simulink model "GenNewRECurrentRef"  (R2016a)
settings: Solver=FixedStepDiscrete  StartTime=0  StopTime=7  FixedStep=0.001  RelTol=1e-3
values from neighbouring files (symbols this model uses):
  beta = 0.9    [base_model_hybrid_REcurrent_init.m]
  deltaTdes = 0.2    [base_model_hybrid_REcurrent_init.m]
  enableMultiplePlateau = 1    [base_model_hybrid_REcurrent_init.m]
  enableUpdateRefUp = 0    [base_model_hybrid_REcurrent_init.m]
  percent_upgain_newiref = 0.1    [base_model_hybrid_REcurrent_init.m]
  t_end = 2.0    (= 2)    [base_model_hybrid_REcurrent_init.m]
  threshold_time_newiref = 0.02    [base_model_hybrid_REcurrent_init.m]
undefined symbols (not defined in the file or in its folder): cq, pwm, rt2, trigger
libraries: powerlib_extras x1
settings Model: ExtModeTrigDuration=2  Creator=hbaole  LastModifiedBy=mateusz
settings DataIOCC: SaveFormat=Array  SignalLoggingSaveFormat=ModelDataLogs  SaveOutput=off  SignalLogging=off  DSMLogging=off  SignalLoggingName=sigsOut
settings OptimizationCC: DefaultParameterBehavior=Inlined  UseDivisionForNetSlopeComputation=on  UseFloatMulNetSlope=on  InlineInvariantSignals=on  EnhancedBackFolding=on  ExpressionDepthLimit=2147483647  StateBitsets=on  DataBitsets=on  EfficientFloat2IntCast=on  OptimizeModelRefInitCode=on  LifeSpan=1  MaxStackSize=64
settings DebuggingCC: RTPrefix=warning  SaveWithParameterizedLinksMsg=none  UnderspecifiedInitializationDetection=Classic  MergeDetectMultiDrivingBlocksExec=none  MultiTaskDSMMsg=warning  MultiTaskCondExecSysMsg=none  FcnCallInpInsideContextMsg=UseLocalSettings  UnconnectedInputMsg=none  UnconnectedOutputMsg=none  UnconnectedLineMsg=none  StateNameClashWarn=warning
settings HardwareCC: TargetBitPerPointer=64  TargetLongLongMode=on  TargetIntDivRoundTo=Zero  TargetEndianess=LittleEndian  TargetWordSize=64  TargetHWDeviceType=MATLAB Host  ProdEqTarget=off
settings ModelReferenceCC: ModelReferenceNumInstancesAllowed=Single  PropagateSignalLabelsOutOfModel=off
settings SFSimCC: SimParseCustomCode=off
settings RTWCC: SystemTargetFile=ert.tlc  GenCodeOnly=on  TemplateMakefile=ert_default_tmf  GenerateReport=on  RTWVerbose=off  RetainRTWFile=on  Toolchain=MinGW64 v4.x | gmake (64-bit Windows)  BuildConfiguration=Specify  IncludeHyperlinkInReport=on  LaunchReport=on  TargetLang=C++  GenerateTraceInfo=on  GenerateTraceReport=on  GenerateTraceReportSl=on  GenerateTraceReportSf=on  GenerateTraceReportEml=on  CheckMdlBeforeBuild=Warning
settings CodeAppCC: ForceParamTrailComments=on  OperatorAnnotations=on  SimulinkDataObjDesc=on  SFDataObjDesc=on  MATLABFcnDesc=on  InsertBlockDesc=on  MATLABSourceComments=on
settings ERTTargetCC: GenerateSampleERTMain=on  MultiInstanceERTCode=on  CodeInterfacePackaging=C++ class  InlinedParameterPlacement=NonHierarchical  RootIOFormat=Structure reference  ERTCustomFileTemplate=example_file_process.tlc
settings ConfigComp: CovModelRefEnable=Off

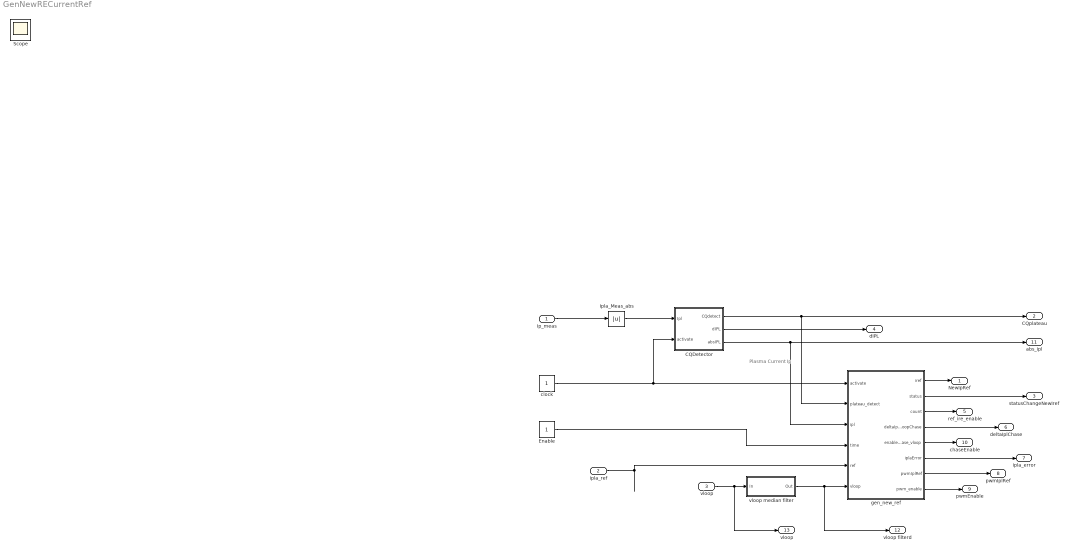
== system GenNewRECurrentRef ==
  note: Plasma Current Ip
  Ip_meas : Inport
  ipla_ref : Inport  Port=2
  vloop : Inport  Port=3
  CQDetector : Subsystem
  Enable : Constant
  Ipla_Meas_abs : Abs
  clock : Constant
  gen_new_ref : Subsystem
  vloop median filter : Subsystem
  NewIpRef : Outport
  CQplateau : Outport  Port=2
  statusChangeNewIref : Outport  Port=3
  dIPL : Outport  Port=4
  ref_ire_enable : Outport  Port=5
  deltaIplChase : Outport  Port=6
  ipla_error : Outport  Port=7
  pwmIplRef : Outport  Port=8
  pwmEnable : Outport  Port=9
  chaseEnable : Outport  Port=10
  abs_ipl : Outport  Port=11
  "vloop filterd " : Outport  Port=12
  "vloop " : Outport  Port=13
  Scope : Scope
  wires:
  CQDetector/1(CQdetect) -> gen_new_ref/2(plateau_detect), CQplateau/1
  CQDetector/2(dIPL) -> dIPL/1
  CQDetector/3(absIPL) -> gen_new_ref/3(ipl), abs_ipl/1
  clock/1 -> CQDetector/2(activate), gen_new_ref/1(activate)
  Ip_meas/1 -> Ipla_Meas_abs/1
  Ipla_Meas_abs/1 -> CQDetector/1(Ipl)
  ipla_ref/1 -> gen_new_ref/5(ref)
  gen_new_ref/1(iref) -> NewIpRef/1
  gen_new_ref/2(status) -> statusChangeNewIref/1
  gen_new_ref/3(count) -> ref_ire_enable/1
  gen_new_ref/4("deltaIplVloopChase ") -> deltaIplChase/1
  gen_new_ref/5(enableChase_vloop) -> chaseEnable/1
  gen_new_ref/6(iplaError) -> ipla_error/1
  gen_new_ref/7(pwmIplRef) -> pwmIplRef/1
  gen_new_ref/8(pwm_enable) -> pwmEnable/1
  Enable/1 -> gen_new_ref/4(time)
  vloop median filter/1(Out) -> "vloop filterd "/1, gen_new_ref/6(vloop)
  vloop/1 -> "vloop "/1, vloop median filter/1(In)

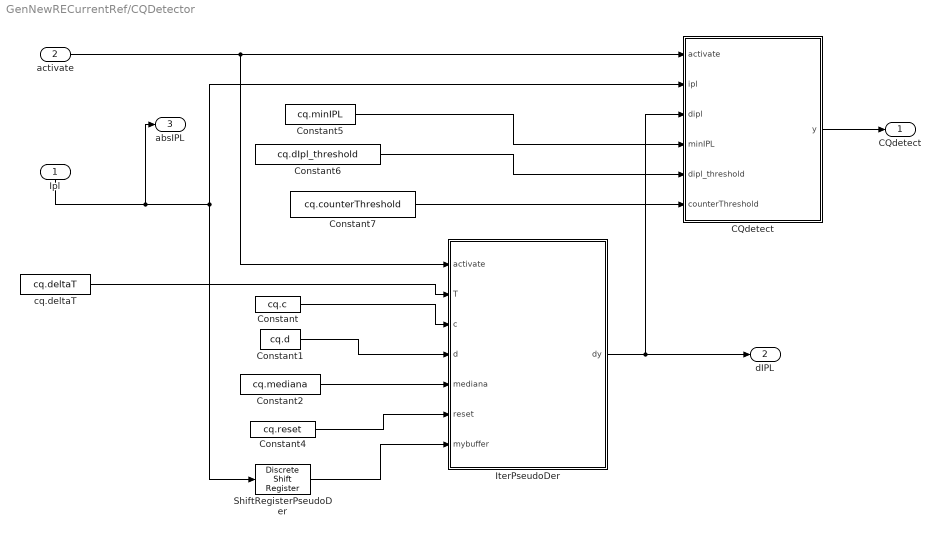
== system GenNewRECurrentRef/CQDetector ==
  Ipl : Inport
  activate : Inport  Port=2
  "CQdetect " : MATLAB Function  TreatAsAtomicUnit=on
  Constant : Constant  Value=cq.c
  Constant1 : Constant  Value=cq.d
  Constant2 : Constant  Value=cq.mediana
  Constant4 : Constant  Value=cq.reset
  Constant5 : Constant  Value=cq.minIPL
  Constant6 : Constant  Value=cq.dIpl_threshold
  Constant7 : Constant  Value=cq.counterThreshold
  IterPseudoDer : MATLAB Function  TreatAsAtomicUnit=on
      settings: RTWSystemCode=Inline
  ShiftRegisterPseudoDer : powerlib_extras/Discrete  Control Blocks/Discrete Shift Register  NSamples=cq.d  InitialValue=0  Ts=rt2.system_period
  cq.deltaT : Constant  Value=cq.deltaT
  CQdetect : Outport
  dIPL : Outport  Port=2
  absIPL : Outport  Port=3
  wires:
  Constant6/1 -> "CQdetect "/5(dipl_threshold)
  activate/1 -> IterPseudoDer/1(activate), "CQdetect "/1(activate)
  Constant5/1 -> "CQdetect "/4(minIPL)
  cq.deltaT/1 -> IterPseudoDer/2(T)
  Constant/1 -> IterPseudoDer/3(c)
  Constant1/1 -> IterPseudoDer/4(d)
  Constant2/1 -> IterPseudoDer/5(mediana)
  Ipl/1 -> absIPL/1, "CQdetect "/2(ipl), ShiftRegisterPseudoDer/1
  "CQdetect "/1(y) -> CQdetect/1
  Constant7/1 -> "CQdetect "/6(counterThreshold)
  IterPseudoDer/1(dy) -> "CQdetect "/3(dipl), dIPL/1
  Constant4/1 -> IterPseudoDer/6(reset)
  ShiftRegisterPseudoDer/1 -> IterPseudoDer/7(mybuffer)

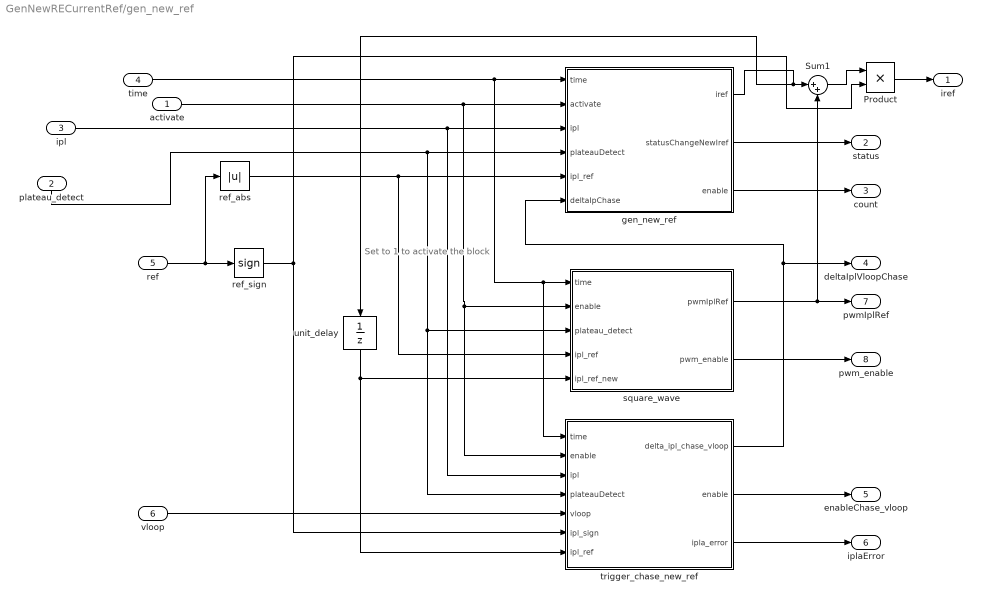
== system GenNewRECurrentRef/gen_new_ref ==
  note: Set to 1 to activate the block
  activate : Inport
  plateau_detect : Inport  Port=2
  ipl : Inport  Port=3
  time : Inport  Port=4
  ref : Inport  Port=5
  vloop : Inport  Port=6
  Product : Product
  Sum1 : Sum  Inputs=|++
  gen_new_ref : Subsystem
  ref_abs : Abs
  ref_sign : Signum
  square_wave : Subsystem
  trigger_chase_new_ref : Subsystem
  unit_delay : UnitDelay  SampleTime=-1
  iref : Outport
  status : Outport  Port=2
  count : Outport  Port=3
  "deltaIplVloopChase " : Outport  Port=4
  enableChase_vloop : Outport  Port=5
  iplaError : Outport  Port=6
  pwmIplRef : Outport  Port=7
  pwm_enable : Outport  Port=8
  wires:
  activate/1 -> trigger_chase_new_ref/2("enable "), square_wave/2("enable "), gen_new_ref/2("activate ")
  ipl/1 -> gen_new_ref/3(ipl), trigger_chase_new_ref/3(ipl)
  ref_abs/1 -> gen_new_ref/5("ipl_ref "), square_wave/4("ipl_ref ")
  time/1 -> square_wave/1(time), trigger_chase_new_ref/1(time), gen_new_ref/1(time)
  ref/1 -> ref_abs/1, ref_sign/1
  ref_sign/1 -> trigger_chase_new_ref/6("ipl_sign "), Product/2
  gen_new_ref/2(statusChangeNewIref) -> status/1
  trigger_chase_new_ref/1(delta_ipl_chase_vloop) -> gen_new_ref/6(deltaIpChase), "deltaIplVloopChase "/1
  gen_new_ref/3(enable) -> count/1
  trigger_chase_new_ref/3(ipla_error) -> iplaError/1
  square_wave/2(pwm_enable) -> pwm_enable/1
  gen_new_ref/1(iref) -> unit_delay/1, Sum1/1
  Sum1/1 -> Product/1
  Product/1 -> iref/1
  vloop/1 -> trigger_chase_new_ref/5(vloop)
  trigger_chase_new_ref/2(enable) -> enableChase_vloop/1
  plateau_detect/1 -> trigger_chase_new_ref/4(plateauDetect), square_wave/3(plateau_detect), gen_new_ref/4(plateauDetect)
  unit_delay/1 -> trigger_chase_new_ref/7("ipl_ref "), square_wave/5(ipl_ref_new)
  square_wave/1(pwmIplRef) -> Sum1/2, pwmIplRef/1

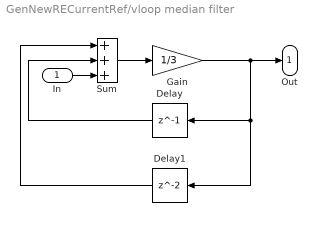
== system GenNewRECurrentRef/vloop median filter ==
  In : Inport
  Delay : Delay  DelayLength=1  InitialCondition=0
  Delay1 : Delay  InitialCondition=0
  Gain : Gain  Gain=1/3
  Sum : Sum  Inputs=|+++  SampleTime=rt2.system_period
  Out : Outport
  wires:
  Gain/1 -> Out/1, Delay1/1, Delay/1
  Delay/1 -> Sum/2
  Sum/1 -> Gain/1
  Delay1/1 -> Sum/1
  In/1 -> Sum/3

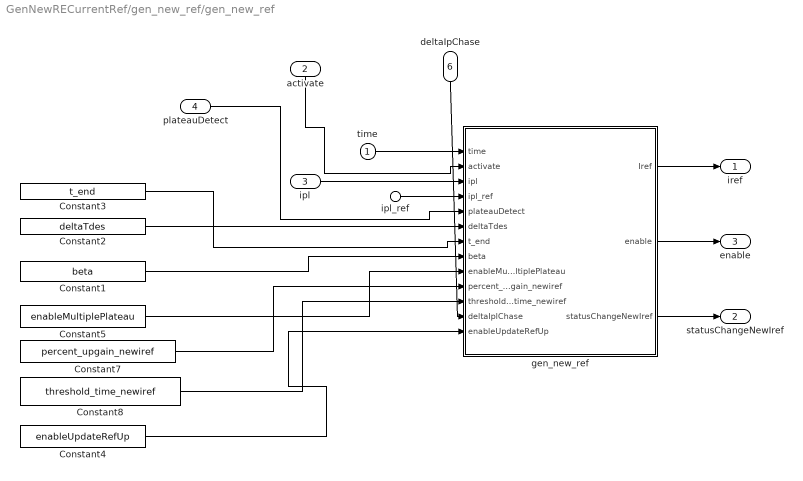
== system GenNewRECurrentRef/gen_new_ref/gen_new_ref ==
  time : Inport
  "activate " : Inport  Port=2
  ipl : Inport  Port=3
  plateauDetect : Inport  Port=4
  "ipl_ref " : Inport  Port=5
  deltaIpChase : Inport  Port=6
  Constant1 : Constant  Value=beta
  Constant2 : Constant  Value=deltaTdes
  Constant3 : Constant  Value=t_end
  Constant4 : Constant  Value=enableUpdateRefUp
  Constant5 : Constant  Value=enableMultiplePlateau
  Constant7 : Constant  Value=percent_upgain_newiref
  Constant8 : Constant  Value=threshold_time_newiref
  gen_new_ref : MATLAB Function  TreatAsAtomicUnit=on
  iref : Outport
  statusChangeNewIref : Outport  Port=2
  enable : Outport  Port=3
  wires:
  plateauDetect/1 -> gen_new_ref/5(plateauDetect)
  gen_new_ref/1(Iref) -> iref/1
  "ipl_ref "/1 -> gen_new_ref/4(ipl_ref)
  gen_new_ref/3(statusChangeNewIref) -> statusChangeNewIref/1
  Constant8/1 -> gen_new_ref/11(threshold_time_newiref)
  Constant7/1 -> gen_new_ref/10(percent_upgain_newiref)
  time/1 -> gen_new_ref/1(time)
  "activate "/1 -> gen_new_ref/2(activate)
  ipl/1 -> gen_new_ref/3(ipl)
  Constant2/1 -> gen_new_ref/6(deltaTdes)
  Constant3/1 -> gen_new_ref/7(t_end)
  gen_new_ref/2(enable) -> enable/1
  Constant5/1 -> gen_new_ref/9(enableMultiplePlateau)
  Constant1/1 -> gen_new_ref/8(beta)
  deltaIpChase/1 -> gen_new_ref/12(deltaIplChase)
  Constant4/1 -> gen_new_ref/13(enableUpdateRefUp)

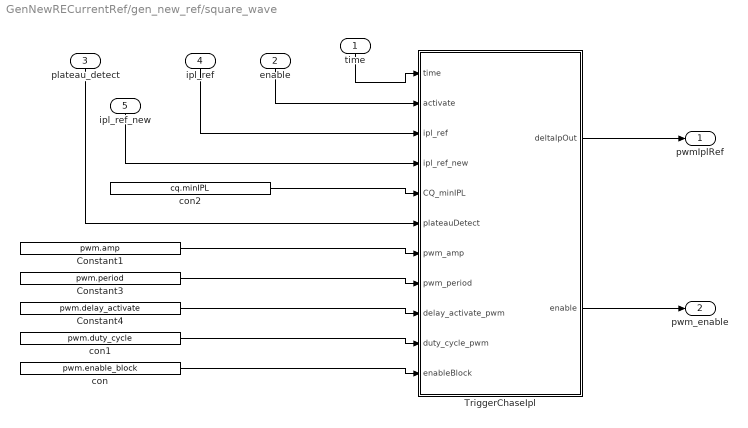
== system GenNewRECurrentRef/gen_new_ref/square_wave ==
  time : Inport
  "enable " : Inport  Port=2
  plateau_detect : Inport  Port=3
  "ipl_ref " : Inport  Port=4
  ipl_ref_new : Inport  Port=5
  Constant1 : Constant  Value=pwm.amp
  Constant3 : Constant  Value=pwm.period
  Constant4 : Constant  Value=pwm.delay_activate
  TriggerChaseIpl : MATLAB Function  TreatAsAtomicUnit=on
  con : Constant  Value=pwm.enable_block
  con1 : Constant  Value=pwm.duty_cycle
  con2 : Constant  Value=cq.minIPL
  pwmIplRef : Outport
  pwm_enable : Outport  Port=2
  wires:
  con/1 -> TriggerChaseIpl/11(enableBlock)
  Constant1/1 -> TriggerChaseIpl/7(pwm_amp)
  TriggerChaseIpl/2(enable) -> pwm_enable/1
  plateau_detect/1 -> TriggerChaseIpl/6(plateauDetect)
  TriggerChaseIpl/1(deltaIpOut) -> pwmIplRef/1
  "enable "/1 -> TriggerChaseIpl/2(activate)
  "ipl_ref "/1 -> TriggerChaseIpl/3(ipl_ref)
  time/1 -> TriggerChaseIpl/1(time)
  Constant3/1 -> TriggerChaseIpl/8(pwm_period)
  Constant4/1 -> TriggerChaseIpl/9(delay_activate_pwm)
  con1/1 -> TriggerChaseIpl/10(duty_cycle_pwm)
  con2/1 -> TriggerChaseIpl/5(CQ_minIPL)
  ipl_ref_new/1 -> TriggerChaseIpl/4(ipl_ref_new)

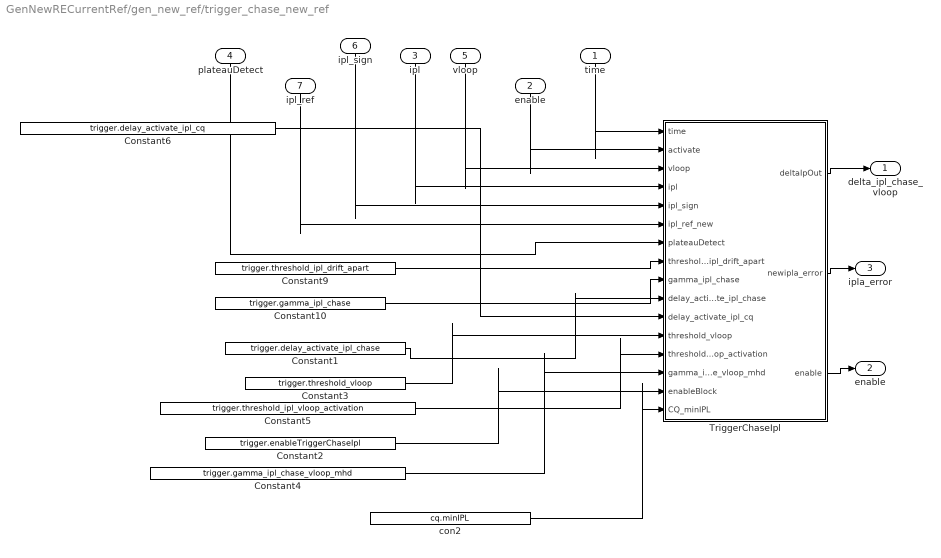
== system GenNewRECurrentRef/gen_new_ref/trigger_chase_new_ref ==
  time : Inport
  "enable " : Inport  Port=2
  ipl : Inport  Port=3
  plateauDetect : Inport  Port=4
  vloop : Inport  Port=5
  "ipl_sign " : Inport  Port=6
  "ipl_ref " : Inport  Port=7
  Constant1 : Constant  Value=trigger.delay_activate_ipl_chase
  Constant10 : Constant  Value=trigger.gamma_ipl_chase
  Constant2 : Constant  Value=trigger.enableTriggerChaseIpl
  Constant3 : Constant  Value=trigger.threshold_vloop
  Constant4 : Constant  Value=trigger.gamma_ipl_chase_vloop_mhd
  Constant5 : Constant  Value=trigger.threshold_ipl_vloop_activation
  Constant6 : Constant  Value=trigger.delay_activate_ipl_cq
  Constant9 : Constant  Value=trigger.threshold_ipl_drift_apart
  TriggerChaseIpl : MATLAB Function  TreatAsAtomicUnit=on
  con2 : Constant  Value=cq.minIPL
  delta_ipl_chase_vloop : Outport
  enable : Outport  Port=2
  ipla_error : Outport  Port=3
  wires:
  ipl/1 -> TriggerChaseIpl/4(ipl)
  time/1 -> TriggerChaseIpl/1(time)
  "ipl_ref "/1 -> TriggerChaseIpl/6(ipl_ref_new)
  Constant10/1 -> TriggerChaseIpl/9(gamma_ipl_chase)
  "enable "/1 -> TriggerChaseIpl/2(activate)
  Constant9/1 -> TriggerChaseIpl/8(threshold_ipl_drift_apart)
  TriggerChaseIpl/1(deltaIpOut) -> delta_ipl_chase_vloop/1
  plateauDetect/1 -> TriggerChaseIpl/7(plateauDetect)
  TriggerChaseIpl/3(enable) -> enable/1
  Constant1/1 -> TriggerChaseIpl/10(delay_activate_ipl_chase)
  Constant2/1 -> TriggerChaseIpl/15(enableBlock)
  TriggerChaseIpl/2(newipla_error) -> ipla_error/1
  vloop/1 -> TriggerChaseIpl/3(vloop)
  "ipl_sign "/1 -> TriggerChaseIpl/5(ipl_sign)
  Constant3/1 -> TriggerChaseIpl/12(threshold_vloop)
  Constant4/1 -> TriggerChaseIpl/14(gamma_ipl_chase_vloop_mhd)
  Constant5/1 -> TriggerChaseIpl/13(threshold_ipl_vloop_activation)
  con2/1 -> TriggerChaseIpl/16(CQ_minIPL)
  Constant6/1 -> TriggerChaseIpl/11(delay_activate_ipl_cq)

== matlab function GenNewRECurrentRef/CQDetector/CQdetect  ==
  data: activate input; ipl input; y output; dipl input; minIPL input; dipl_threshold input; counterThreshold input
function y = cq_detect(activate, ipl, dipl, minIPL, dipl_threshold, counterThreshold)
%% CurrentQuench and RE palteau detection
% INPUT:
%          activate = boolean var for eneabled the alghoritm
%                      0 : active
%                      1 : non active
%           ipl = absolute value of the  plasma current
%           dipl, minIPL, dipl_threshold, counterThreshold : min
%
% OUTPUT:  y in R
%         -1 : detection non active
%          0 : detection active
%          1 : CQ detect
%          2 : RE palteau detect
%%

persistent  startDetection;

if(activate)
    if(isempty(startDetection))
        startDetection = 0;
    end
    
    %STEP1: FIND CQ
    if( ipl >= minIPL)
        
        if( dipl <= dipl_threshold  && mod(startDetection,2)  == 0)
            startDetection = startDetection+1;
        end
        
        if( dipl >=  dipl_threshold  && mod(startDetection,2) == 1)
            startDetection = startDetection+1;
        end
        
    else
        
        if(startDetection > 0)
            startDetection =-1;
        end
        
    end
    
    y = startDetection;
    
else
    y = -2;
end

== matlab function GenNewRECurrentRef/CQDetector/IterPseudoDer ==
  data: activate input; T input; c input; d input; mediana input; reset input; dy output; mybuffer input
function dy = iter_pseudo_der_function(activate,T,c,d,mediana,reset,mybuffer)

 if activate==1 && reset==0
     
     if(mediana==1)
         temp1 = 0;
         temp2 = 0;
         
         % La mediana non compila con rtwbuild,
         % dobbiamo indagare perche' per il momento commentata
         %temp1 = median(mybuffer(1:c));
         %temp2 = median(mybuffer(d-c+1:d));
     else
         temp1 = 0;
        for k=1:c
            temp1 = temp1 + mybuffer(k);
        end
        temp1 = temp1/c;
        
         temp2 = 0;
        for k=d-c+1:d
            temp2 = temp2 + mybuffer(k);
        end
        
        temp2 = temp2/c;
     end
     
     dy = (temp1-temp2) / (T*(d-c));
     
else
     dy = 0;
end



end

== matlab function GenNewRECurrentRef/gen_new_ref/gen_new_ref/gen_new_ref ==
  data: time input; activate input; ipl input; Iref output; ipl_ref input; plateauDetect input; deltaTdes input; t_end input; beta input; enable output; enableMultiplePlateau input; percent_upgain_newiref input; threshold_time_newiref input; statusChangeNewIref output; deltaIplChase input; enableUpdateRefUp input
 function [Iref, enable, statusChangeNewIref] = ire_ref(time, activate, ipl, ipl_ref, plateauDetect, deltaTdes ,...
    t_end ,beta, enableMultiplePlateau,...
    percent_upgain_newiref,threshold_time_newiref, deltaIplChase, enableUpdateRefUp )
%% COMPUTE NEW REFERENCE FOR RUNAWAY ELECTRON CURRENT BEAM
% INPUT:
%           time     =
%           activate = boolean var for eneabled the alghoritm
%                      0 : active
%                      1 : non active
%           ipl      = absolute value of the  plasma current
%           dipl     = derivative of abs(ipl)
%           ipl_ref  = prep_reference
%           plateauDetect =
%           deltaTdes     =
%           t_end         =
%           beta          =
%
% OUTPUT:  y in R
%          y is the new reference for the ipl
%%

persistent  enableCurrentDecay Iptpl tpl Ireftpl counter;

Iref = ipl_ref;
enable = 0;
statusChangeNewIref= 0;
if(activate)
    if(isempty(enableCurrentDecay))
        enableCurrentDecay = 0;
        Iptpl = 0;
        tpl = 0;
        Ireftpl = 0;
        counter = 0;
    end
    
    if(plateauDetect >=2)
        
        if( mod(plateauDetect,2) == 0 && ...
                enableCurrentDecay == (plateauDetect/2-1))
            % 2 && 0, 4 && 1 , 6 && 2 ecc..
            if(plateauDetect == 2 || enableMultiplePlateau == 1)
                %enableMultiplePlateau
                enableCurrentDecay = enableCurrentDecay + 1 ;
                %init var
                Iptpl   = ipl;
                if(enableCurrentDecay == 1)
                    %only ones
                    Ireftpl = ipl_ref;
                end
                tpl     = time;
                counter = 0;
            end
        end
        
        
        
        
    end
    
    
    
    if( enableCurrentDecay >= 1 )
        
        if(counter == 0)
            if(enableCurrentDecay == 1)
                Ireftpl = ipl_ref;
            end
        else
            
            %update program down
            newipla_error = (ipl-Ireftpl);
            
            %update program up
            if(enableUpdateRefUp == 1)
                if (newipla_error >= 0 && (t_end-time) >= threshold_time_newiref)
                    %update Iref_linear
                    Iptpl = ipl+(ipl*percent_upgain_newiref);
                    statusChangeNewIref=statusChangeNewIref + 1;
                end
            end
            
            
            
            % compute linear slop
            t_final = min(deltaTdes , t_end - tpl);
            alpha = Iptpl/(t_final);
            Iref_linear = (Iptpl) - alpha*(time-tpl) + deltaIplChase;
            % compute exp decay
            Ireftpl = (beta)*Ireftpl+(1-beta)*Iref_linear;
            
        end
        counter = counter +1;
        Iref =  Ireftpl;
        
        if(Iref <0) % disable
            enableCurrentDecay = -1;
        end
        
    end
    
    if(enableCurrentDecay == -1)
        Iref = 0;
    end
    

    
    enable = enableCurrentDecay;
    
end

== matlab function GenNewRECurrentRef/gen_new_ref/square_wave/TriggerChaseIpl ==
  data: deltaIpOut output; time input; activate input; ipl_ref input; ipl_ref_new input; CQ_minIPL input; plateauDetect input; enable output; pwm_amp input; pwm_period input; delay_activate_pwm input; duty_cycle_pwm input; enableBlock input
function [deltaIpOut, enable]  = square_wave(time, activate, ipl_ref, ipl_ref_new, CQ_minIPL, plateauDetect,...
    pwm_amp, pwm_period, delay_activate_pwm, duty_cycle_pwm, enableBlock)
%% COMPUTE PWM SIGNAL
% INPUT:
%           time     =
%           activate = boolean var for eneabled the alghoritm
%                      0 : active
%                      1 : non active
%           ipl      = absolute value of the  plasma current
%           dipl     = derivative of abs(ipl)
%           ipl_ref  = prep_reference
%
% OUTPUT:  y in R
%          y is the new reference for the ipl
%%

persistent    deltaIpl  startTime plateauDetectOld enableChase waitTime;

enable = 0;
deltaIpOut = 0;

if(activate && enableBlock)
    
    if(isempty(deltaIpl))
        deltaIpl = 0;
        waitTime = 0;
        enableChase = 0;
        plateauDetectOld= 0;
        startTime = 0;
    end
    
    
    % cq condition
    if(mod(plateauDetect,2) == 0 && plateauDetectOld ~= plateauDetect && plateauDetect >= 2)
        waitTime = time;
        enableChase = 1;
    end
    plateauDetectOld = plateauDetect;
    
    
    if((time-waitTime) >= delay_activate_pwm && enableChase >= 1 && plateauDetect >= 2)
        
        if(enableChase == 1)
            startTime =time;
        end        
        
        pwmTime = time-startTime;
        
        if( pwmTime < pwm_period )
            deltaIpl = -pwm_amp;
            enableChase = 2;
            if( pwmTime < pwm_period*duty_cycle_pwm )
                deltaIpl = pwm_amp;
                enableChase = 3;
            end
        else
            %reset pwmTime
            enableChase = 1;
        end   
    else
         deltaIpl = 0.0;          
    end
    

    if( pwm_amp > (ipl_ref_new-CQ_minIPL) || mod(plateauDetect,2) ~= 0)
        deltaIpl = 0;
        enableChase = 0;
    end
    
    
    enable = enableChase;
    deltaIpOut =  deltaIpl;
   
end

== matlab function GenNewRECurrentRef/gen_new_ref/trigger_chase_new_ref/TriggerChaseIpl ==
  data: deltaIpOut output; newipla_error output; time input; activate input; vloop input; ipl input; ipl_sign input; ipl_ref_new input; plateauDetect input; enable output; threshold_ipl_drift_apart input; gamma_ipl_chase input; delay_activate_ipl_chase input; delay_activate_ipl_cq input; threshold_vloop input; threshold_ipl_vloop_activation input; gamma_ipl_chase_vloop_mhd input; enableBlock input; CQ_minIPL input
function [deltaIpOut, newipla_error, enable]  = chase_ipl_ref(time, activate, vloop, ipl, ipl_sign, ipl_ref_new, plateauDetect,...
                                                            threshold_ipl_drift_apart, gamma_ipl_chase, delay_activate_ipl_chase,delay_activate_ipl_cq,...
                                                            threshold_vloop,threshold_ipl_vloop_activation, gamma_ipl_chase_vloop_mhd, enableBlock,CQ_minIPL)

%% COMPUTE NEW REFERENCE FOR RUNAWAY ELECTRON CURRENT BEAM WHEN ref and ipl are fall apart
% INPUT:
%           time     = 
%           activate = boolean var for eneabled the alghoritm
%                      0 : active
%                      1 : non active
%           ipl                         = absolute value of the  plasma current
%           dipl                        = derivative of abs(ipl)
%           ipl_ref                     = prep_reference
%           plateauDetect = 2,4,6...    =
%           threshold_ipl_fall_apart    =   
%           gamma_ipl_chase: 
%           delay_activate_ipl_chase:
%           enablePwm = 
% OUTPUT:  deltaIpOut: 
%          newipla_error: error 
%          enable
%%

persistent    deltaIpl   plateauDetectOld enableChase waitTime waitTimeChase;

enable = 0;
deltaIpOut = 0;
newipla_error = (ipl-ipl_ref_new);

if(activate && enableBlock)
    
    if(isempty(deltaIpl))
        deltaIpl = 0;
        waitTime = 0;
        enableChase = 0;
        plateauDetectOld= 0;
        waitTimeChase = 0.0;
    end
    
    if(plateauDetect >= 1)
        % cq condition
        if(mod(plateauDetect,2) == 0 && plateauDetectOld ~= plateauDetect)
            waitTime = time;
            enableChase = 1;
        end
        plateauDetectOld = plateauDetect;
        
        
        if(((time-waitTime) >= delay_activate_ipl_cq && (time-waitTimeChase) >=delay_activate_ipl_chase) && enableChase == 1 && ipl_ref_new >= CQ_minIPL)
            
            
            if((abs(newipla_error) >= threshold_ipl_drift_apart || -vloop*ipl_sign >= threshold_vloop) && mod(plateauDetect,2) == 0)
                enable = 1;
                newDelta = 0.0;
                
                if((abs(newipla_error) >= threshold_ipl_drift_apart))
                    newDelta = gamma_ipl_chase*newipla_error; 
                end
                
                %if vloop is due to mhd resistivity then 
                if( -vloop*ipl_sign >= threshold_vloop && newipla_error <= threshold_ipl_vloop_activation)
                    newDelta = -gamma_ipl_chase_vloop_mhd*ipl;
                end
                
                
                
                deltaIpl =  deltaIpl+newDelta;                
                waitTimeChase = time;
                
            end
            
            
            
        end
    end
    
    
    deltaIpOut =  deltaIpl;
    
end
